simulink model "TESTINOUT"  (Simulink 6.5)
settings: Solver=ode45  StartTime=0.0  StopTime=10.0  RelTol=1e-3
libraries: cdsFilt x1, dac x1, simulink x1, cdsParameters x1
settings Model: Creator=jay  LastModifiedBy=jay

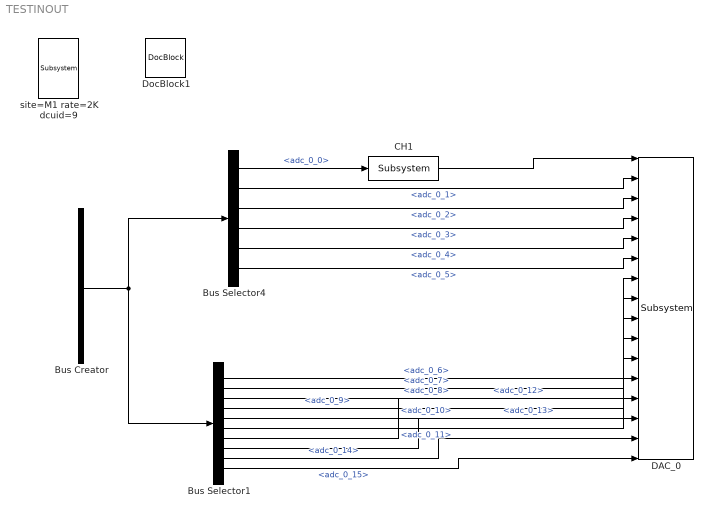
== system TESTINOUT ==
  Bus Creator : BusCreator  Tag=adc_0  Description=|  Inputs='adc_0_0','adc_0_1','adc_0_2','adc_0_3','adc_0_4','adc_0_5','adc_0_6','adc_0_7','adc_0_8','adc_0_9','adc_0_10','adc_0_11','adc_0_12','adc_0_13','adc_0_14','adc_0_15','adc_0_16','adc_0_17','adc_0_18','adc_0_19','adc_0_20','adc_0_21','adc_0_22','adc_0_23','adc_0_24','adc_0_25','adc_0_26','adc_0_27','adc_0_28','adc_0_29','adc_0_30','adc_0_31'
      | PCI66-16AI64SSA
      | 40Vp-p, 16-bit, 610uV/count
      settings: AttributesFormatString=%<Description>\n%<Tag>
  Bus Selector1 : BusSelector  OutputSignals=adc_0_6,adc_0_7,adc_0_8,adc_0_9,adc_0_10,adc_0_11,adc_0_12,adc_0_13,adc_0_14,adc_0_15
  Bus Selector4 : BusSelector  OutputSignals=adc_0_0,adc_0_1,adc_0_2,adc_0_3,adc_0_4,adc_0_5
  CH1 : cdsFilt/Subsystem  Tag=cdsFilt  Description=|  SystemSampleTime=-1
      | Purpose:                                                                                                                                                                                                                                  
      | Standard CDS IIR filter module.                                                                                                                                                                                                           
      |                                                                                                                                                                                                                                           
      | Operation:                                                                                                                                                                                                                                
      | Consists of 10 second order section IIR filters, plus a ramped gain stage. In FE code, also provides pre-defined test points and excitation channel inputs. The filter coefficients are defined in the LIGO system using the 'foton' tool.
      |                                                                                                                                                                                                                                           
      | Usage:                                                                                                                                                                                                                                    
      | Name the part with the desired filter module name.
      settings: AttributesFormatString=%<Tag>
  DAC_0 : dac/Subsystem  Tag=dac_0  Description=|  SystemSampleTime=-1
      | PCI66-16AO16
      | 20Vp-p, 16-bit, 305uV/count
      settings: AttributesFormatString=%<Description>
  DocBlock1 : simulink/Model-Wide Utilities/DocBlock  Tag=SW Install  SystemSampleTime=-1  DocumentType=Text
      settings: AttributesFormatString=%<Tag>
  site=M1 rate=2K dcuid=9 : cdsParameters/Subsystem  Tag=cdsParameters  SystemSampleTime=-1
      settings: AttributesFormatString=%<Tag>
  wires:
  Bus Selector4/1 -> CH1/1  "<adc_0_0>"
  Bus Selector4/2 -> DAC_0/2  "<adc_0_1>"
  Bus Selector4/3 -> DAC_0/3  "<adc_0_2>"
  Bus Selector4/4 -> DAC_0/4  "<adc_0_3>"
  Bus Selector4/5 -> DAC_0/5  "<adc_0_4>"
  Bus Selector4/6 -> DAC_0/6  "<adc_0_5>"
  Bus Selector1/1 -> DAC_0/7  "<adc_0_6>"
  Bus Creator/1 -> Bus Selector4/1, Bus Selector1/1
  CH1/1 -> DAC_0/1
  Bus Selector1/2 -> DAC_0/8  "<adc_0_7>"
  Bus Selector1/3 -> DAC_0/9  "<adc_0_8>"
  Bus Selector1/4 -> DAC_0/10  "<adc_0_9>"
  Bus Selector1/5 -> DAC_0/11  "<adc_0_10>"
  Bus Selector1/6 -> DAC_0/12  "<adc_0_11>"
  Bus Selector1/7 -> DAC_0/13  "<adc_0_12>"
  Bus Selector1/8 -> DAC_0/14  "<adc_0_13>"
  Bus Selector1/9 -> DAC_0/15  "<adc_0_14>"
  Bus Selector1/10 -> DAC_0/16  "<adc_0_15>"
